simulink model "Bug_checking"  (R2018b)
settings: Solver=FixedStepAuto  StartTime=0.0  StopTime=10.0  FixedStep=simParams.sample_time_s  RelTol=1e-3
libraries: CDH_command_lib x1, FSW_Lib x1
settings Model: Creator=colem  LastModifiedBy=colem

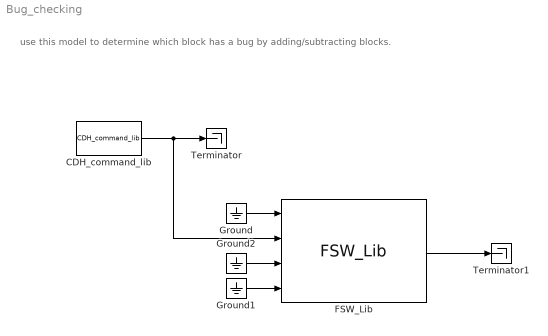
== system Bug_checking ==
  note: use this model to determine which block has a bug by adding/subtracting blocks.
  CDH_command_lib : CDH_command_lib/CDH_command_lib  SystemSampleTime=-1
  FSW_Lib : FSW_Lib/FSW_Lib  SystemSampleTime=-1
  Ground : Ground
  Ground1 : Ground
  Ground2 : Ground
  Terminator : Terminator
  Terminator1 : Terminator
  wires:
  CDH_command_lib/1 -> FSW_Lib/2, Terminator/1
  Ground/1 -> FSW_Lib/1
  Ground2/1 -> FSW_Lib/3
  Ground1/1 -> FSW_Lib/4
  FSW_Lib/1 -> Terminator1/1
